simulink model "JKFF_CMOS"  (R2024b)
settings: Solver=VariableStepAuto  StartTime=0.0  StopTime=1e-6  RelTol=1e-3
libraries: ee_lib x22, fl_lib x10, nesl_utility x6
settings Model: Creator=Soochan Kim  LastModifiedBy=Soochan Kim

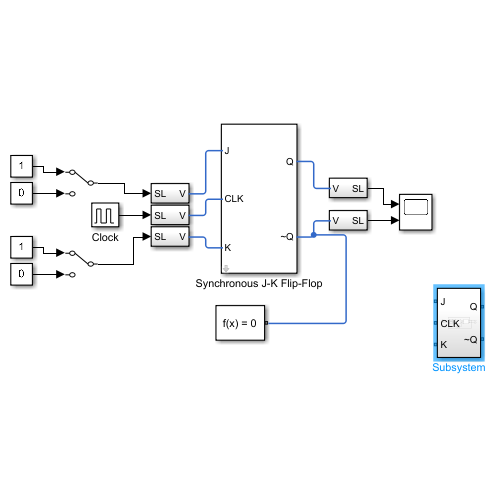
[thumbnail: Simulink's stored preview of the top-level diagram]
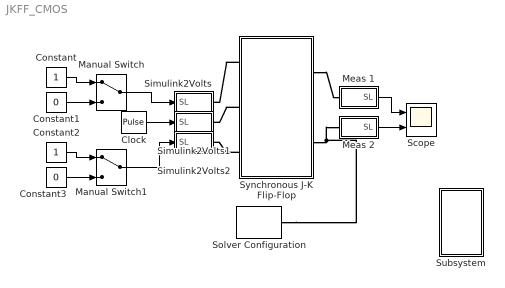
== system JKFF_CMOS ==
  Clock : DiscretePulseGenerator  PulseType=Time based  Amplitude=10  Period=2e-7  PulseWidth=50  PhaseDelay=0.5e-7
  Constant : Constant
  Constant1 : Constant  Value=0
  Constant2 : Constant
  Constant3 : Constant  Value=0
  Manual Switch : ManualSwitch
  Manual Switch1 : ManualSwitch
  Meas 1 : Subsystem
  Meas 2 : Subsystem
  Scope : Scope  NumInputPorts=2
  Simulink2Volts : Subsystem
  Simulink2Volts1 : Subsystem
  Simulink2Volts2 : Subsystem
  Solver Configuration : nesl_utility/Solver Configuration  PhysicalDomain=network_engine_domain  SubClassName=solver  LeftPortType=input  RightPortType=generic  Tones=[]  Harmonics=[]  SimulateNoise=off  Profile=off  UseLocalSampling=off  EnableSwitchedLinearOptims=on  FrequencyDomain=off  UseCCode=off  RelTol=0.001  AbsTol=0.001  MinStep=1e-09  ToWorkspace=off  RevertToSquareIcSolve=off  NumHomotopyIterations=100  PhasorMode=off  PhasorModeNumHarmonics=1  ConsistencySolver=NEWTON_XTOL_AFTER_FTOL  IndexReductionMethod=DerivativeReplacement  DoDC=off  ResidualTolerance=1e-09  ConsistencyTolSource=GLOBAL  ConsistencyAbsTol=0.001  ConsistencyRelTol=0.001  ConsistencyTolFactor=0.001  UseLocalSolver=off  LocalSolverChoice=NE_BACKWARD_EULER_ADVANCER  ResolveIndetEquations=on  FunctionEvalNumThread=1  LocalSolverSampleTime=0.001  DoFixedCost=off  MaxNonlinIter=3  MaxModeIter=2  ComputeImpulses=off  ImpulseIterations=2  LinearAlgebra=auto  LinearAlgebraNumThread=0  EquationFormulation=NE_TIME_EF  DelaysMemoryBudget=1024  AutomaticFiltering=on  FilteringTimeConstant=0.001  PartitionStorageMethod=AS_NEEDED  PartitionMemoryBudget=1024  PartitionMethod=ROBUST  MultibodyUseLocalSolver=off  MultibodyLocalSolverChoice=ODE1  MultibodyLocalSolverSampleTime=0.001
  Subsystem : Subsystem
  Synchronous J-K Flip-Flop : Subsystem  Tag=PublishSubsystem  mask(Synchronous J-K Flip-Flop){C_iss=0.1, t_p=1e-9, V_DD=10, R=450, state=High}
      mask prompts: C_iss "Gate input capacitance (pF)"; t_p "Gate propagation delay (s)"; V_DD "Supply voltage (V)"; R "Gate effective output resistance (ohms)"; state "Initial output"
      mask help: Behavioral model of a synchronous J-K flip-flop built from Simscape(TM) Electrical(TM) library components.
      mask init:
      | h = get_param(gcb,'Handle');
      | SR1 = sprintf('S-R Clocked\nFlip-Flop 1');
      | SR2 = sprintf('S-R Clocked\nFlip-Flop 2');
      | blk_path = [get_param(h,'Parent') '/' get_param(h,'Name')];
      | set_param([blk_path '/' SR1 '/NAND 3'],'output_state',num2str(state))
      | set_param([blk_path '/' SR2 '/NAND 3'],'output_state',num2str(state))
      | set_param([blk_path '/' SR1 '/NAND 4'],'output_state',num2str(3-state))
      | set_param([blk_path '/' SR2 '/NAND 4'],'output_state',num2str(3-state))
      mask TypeOptions state: Low | High
  wires:
  Constant/1 -> Manual Switch/1
  Constant1/1 -> Manual Switch/2
  Constant3/1 -> Manual Switch1/2
  Constant2/1 -> Manual Switch1/1
  Manual Switch/1 -> Simulink2Volts/1(SL)
  Manual Switch1/1 -> Simulink2Volts2/1(SL)
  Meas 1/1(SL) -> Scope/1
  Meas 2/1(SL) -> Scope/2
  Clock/1 -> Simulink2Volts1/1(SL)
  connections:
  Synchronous J-K Flip-Flop/RConn1 -- Meas 1/LConn1
  Synchronous J-K Flip-Flop/RConn2 -- Solver Configuration/RConn1 -- Meas 2/LConn1
  Synchronous J-K Flip-Flop/LConn1 -- Simulink2Volts/RConn1
  Synchronous J-K Flip-Flop/LConn2 -- Simulink2Volts1/RConn1
  Synchronous J-K Flip-Flop/LConn3 -- Simulink2Volts2/RConn1

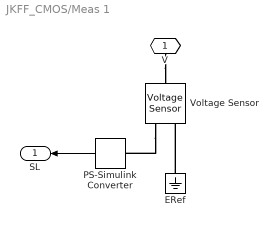
== system JKFF_CMOS/Meas 1 ==
  ERef : fl_lib/Electrical/Electrical Elements/Electrical Reference
  PS-Simulink Converter : nesl_utility/PS-Simulink Converter  PhysicalDomain=network_engine_domain  SubClassName=ps_output  LeftPortType=input  RightPortType=output  PseudoPeriodic=off  Frequencies=[]  VectorFormat=1-D array  Unit=V  AffineConversion=off
  Voltage Sensor : fl_lib/Electrical/Electrical Sensors/Voltage Sensor
  V : PMIOPort  Side=Left
  SL : Outport  VectorParamsAs1DForOutWhenUnconnected=off
  wires:
  PS-Simulink Converter/1 -> SL/1
  connections:
  V/RConn1 -- Voltage Sensor/LConn1
  ERef/LConn1 -- Voltage Sensor/RConn2
  Voltage Sensor/RConn1 -- PS-Simulink Converter/LConn1

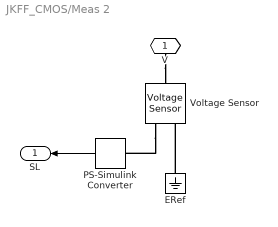
== system JKFF_CMOS/Meas 2 ==
  ERef : fl_lib/Electrical/Electrical Elements/Electrical Reference
  PS-Simulink Converter : nesl_utility/PS-Simulink Converter  PhysicalDomain=network_engine_domain  SubClassName=ps_output  LeftPortType=input  RightPortType=output  PseudoPeriodic=off  Frequencies=[]  VectorFormat=1-D array  Unit=V  AffineConversion=off
  Voltage Sensor : fl_lib/Electrical/Electrical Sensors/Voltage Sensor
  V : PMIOPort  Side=Left
  SL : Outport  VectorParamsAs1DForOutWhenUnconnected=off
  wires:
  PS-Simulink Converter/1 -> SL/1
  connections:
  V/RConn1 -- Voltage Sensor/LConn1
  ERef/LConn1 -- Voltage Sensor/RConn2
  Voltage Sensor/RConn1 -- PS-Simulink Converter/LConn1

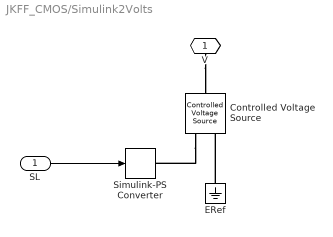
== system JKFF_CMOS/Simulink2Volts ==
  SL : Inport
  Controlled Voltage Source : fl_lib/Electrical/Electrical Sources/Controlled Voltage Source
  ERef : fl_lib/Electrical/Electrical Elements/Electrical Reference
  Simulink-PS Converter : nesl_utility/Simulink-PS Converter  PhysicalDomain=network_engine_domain  SubClassName=ps_input  LeftPortType=input  RightPortType=output  PseudoPeriodic=off  Frequencies=[]  NoiseDistribution=none  NoiseParameters=[]  Unit=V  AffineConversion=off  FilteringAndDerivatives=zero  SimscapeFilterOrder=1  InputFilterTimeConstant=.001  UdotUserProvided=0
  V : PMIOPort  Side=Right
  wires:
  SL/1 -> Simulink-PS Converter/1
  connections:
  V/RConn1 -- Controlled Voltage Source/LConn1
  ERef/LConn1 -- Controlled Voltage Source/RConn2
  Controlled Voltage Source/RConn1 -- Simulink-PS Converter/RConn1

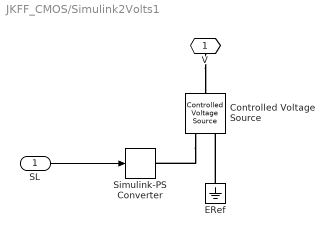
== system JKFF_CMOS/Simulink2Volts1 ==
  SL : Inport
  Controlled Voltage Source : fl_lib/Electrical/Electrical Sources/Controlled Voltage Source
  ERef : fl_lib/Electrical/Electrical Elements/Electrical Reference
  Simulink-PS Converter : nesl_utility/Simulink-PS Converter  PhysicalDomain=network_engine_domain  SubClassName=ps_input  LeftPortType=input  RightPortType=output  PseudoPeriodic=off  Frequencies=[]  NoiseDistribution=none  NoiseParameters=[]  Unit=V  AffineConversion=off  FilteringAndDerivatives=zero  SimscapeFilterOrder=1  InputFilterTimeConstant=.001  UdotUserProvided=0
  V : PMIOPort  Side=Right
  wires:
  SL/1 -> Simulink-PS Converter/1
  connections:
  V/RConn1 -- Controlled Voltage Source/LConn1
  ERef/LConn1 -- Controlled Voltage Source/RConn2
  Controlled Voltage Source/RConn1 -- Simulink-PS Converter/RConn1

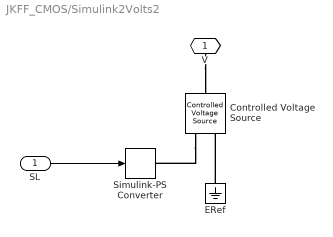
== system JKFF_CMOS/Simulink2Volts2 ==
  SL : Inport
  Controlled Voltage Source : fl_lib/Electrical/Electrical Sources/Controlled Voltage Source
  ERef : fl_lib/Electrical/Electrical Elements/Electrical Reference
  Simulink-PS Converter : nesl_utility/Simulink-PS Converter  PhysicalDomain=network_engine_domain  SubClassName=ps_input  LeftPortType=input  RightPortType=output  PseudoPeriodic=off  Frequencies=[]  NoiseDistribution=none  NoiseParameters=[]  Unit=V  AffineConversion=off  FilteringAndDerivatives=zero  SimscapeFilterOrder=1  InputFilterTimeConstant=.001  UdotUserProvided=0
  V : PMIOPort  Side=Right
  wires:
  SL/1 -> Simulink-PS Converter/1
  connections:
  V/RConn1 -- Controlled Voltage Source/LConn1
  ERef/LConn1 -- Controlled Voltage Source/RConn2
  Controlled Voltage Source/RConn1 -- Simulink-PS Converter/RConn1

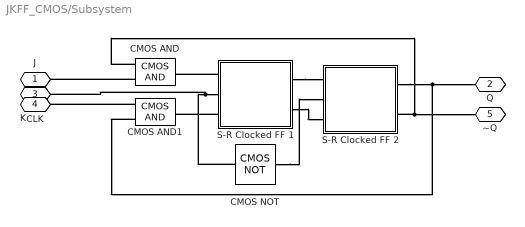
== system JKFF_CMOS/Subsystem ==
  CMOS AND : ee_lib/Integrated Circuits/Logic/CMOS AND  V_IL=2 V  V_IH=3 V  C_IN=5 pF  output_type=ee.enum.ic.outputType.linear  V_OL=0 V  V_OH=5 V  V_CC=5 V  V_meas=5 V  R_OUT=25 Ohm  R_OH=[25, 250] Ohm  I_OH=63 mA  R_OL=[30, 800] Ohm  I_OL=-45 mA  Delay=25 ns  Ron=5 Ohm  Vf=0.6 V  output_state=ee.enum.ic.initialState.low
      settings: InternalSimscapePortConfiguration="{\"Bottom\":[],\"Left\":[{\"id\":\"A\",\"label\":\"\",\"type\":\"foundation.electrical.electrical\"},{\"id\":\"B\",\"label\":\"\",\"type\":\"foundation.electrical.electrical\"}],\"Right\":[{\"id\":\"J\",\"label\":\"\",\"type\":\"foundation.electrical.electrical\"}],\"Top\":[]}"
  CMOS AND1 : ee_lib/Integrated Circuits/Logic/CMOS AND  V_IL=2 V  V_IH=3 V  C_IN=5 pF  output_type=ee.enum.ic.outputType.linear  V_OL=0 V  V_OH=5 V  V_CC=5 V  V_meas=5 V  R_OUT=25 Ohm  R_OH=[25, 250] Ohm  I_OH=63 mA  R_OL=[30, 800] Ohm  I_OL=-45 mA  Delay=25 ns  Ron=5 Ohm  Vf=0.6 V  output_state=ee.enum.ic.initialState.low
      settings: InternalSimscapePortConfiguration="{\"Bottom\":[],\"Left\":[{\"id\":\"A\",\"label\":\"\",\"type\":\"foundation.electrical.electrical\"},{\"id\":\"B\",\"label\":\"\",\"type\":\"foundation.electrical.electrical\"}],\"Right\":[{\"id\":\"J\",\"label\":\"\",\"type\":\"foundation.electrical.electrical\"}],\"Top\":[]}"
  CMOS NOT : ee_lib/Integrated Circuits/Logic/CMOS NOT  V_IL=2 V  V_IH=3 V  C_IN=5 pF  output_type=ee.enum.ic.outputType.linear  V_OL=0 V  V_OH=5 V  V_CC=5 V  V_meas=5 V  R_OUT=25 Ohm  R_OH=[25, 250] Ohm  I_OH=63 mA  R_OL=[30, 800] Ohm  I_OL=-45 mA  Delay=25 ns  Ron=5 Ohm  Vf=0.6 V  output_state=ee.enum.ic.initialState.low
      settings: InternalSimscapePortConfiguration="{\"Bottom\":[],\"Left\":[{\"id\":\"A\",\"label\":\"\",\"type\":\"foundation.electrical.electrical\"}],\"Right\":[{\"id\":\"J\",\"label\":\"\",\"type\":\"foundation.electrical.electrical\"}],\"Top\":[]}"
  S-R Clocked FF 1 : Subsystem
  S-R Clocked FF 2 : Subsystem
  J : PMIOPort  Side=Left
  Q : PMIOPort  Port=2  Side=Right
  CLK : PMIOPort  Port=3  Side=Left
  K : PMIOPort  Port=4  Side=Left
  ~Q : PMIOPort  Port=5  Side=Right
  connections:
  CMOS AND/LConn1 -- S-R Clocked FF 2/RConn2 -- ~Q/RConn1
  S-R Clocked FF 1/LConn3 -- CMOS AND1/RConn1
  S-R Clocked FF 1/RConn1 -- S-R Clocked FF 2/LConn1
  S-R Clocked FF 1/RConn2 -- S-R Clocked FF 2/LConn3
  CMOS NOT/RConn1 -- S-R Clocked FF 2/LConn2
  CMOS AND1/LConn2 -- S-R Clocked FF 2/RConn1 -- Q/RConn1
  CMOS AND1/LConn1 -- K/RConn1
  S-R Clocked FF 1/LConn1 -- CMOS AND/RConn1
  S-R Clocked FF 1/LConn2 -- CMOS NOT/LConn1 -- CLK/RConn1
  CMOS AND/LConn2 -- J/RConn1

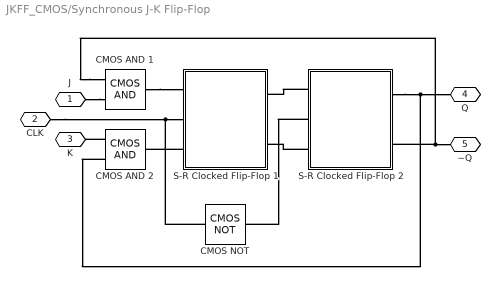
== system JKFF_CMOS/Synchronous J-K Flip-Flop ==
  CMOS AND 1 : ee_lib/Integrated Circuits/Logic/CMOS AND  V_IL=0.4*V_DD V  V_IH=0.6*V_DD V  C_IN=C_iss pF  output_type=1  V_OL=0 V  V_OH=V_DD V  V_CC=5 V  V_meas=5 V  R_OUT=R Ohm  R_OH=[ 25 250 ] Ohm  I_OH=63 mA  R_OL=[ 30 800 ] Ohm  I_OL=-45 mA  Delay=t_p s  Ron=5 Ohm  Vf=0.6 V  output_state=1
      settings: InternalSimscapePortConfiguration="{\"Bottom\":[],\"Left\":[{\"id\":\"A\",\"label\":\"\",\"type\":\"foundation.electrical.electrical\"},{\"id\":\"B\",\"label\":\"\",\"type\":\"foundation.electrical.electrical\"}],\"Right\":[{\"id\":\"J\",\"label\":\"\",\"type\":\"foundation.electrical.electrical\"}],\"Top\":[]}"
  CMOS AND 2 : ee_lib/Integrated Circuits/Logic/CMOS AND  V_IL=0.4*V_DD V  V_IH=0.6*V_DD V  C_IN=C_iss pF  output_type=1  V_OL=0 V  V_OH=V_DD V  V_CC=5 V  V_meas=5 V  R_OUT=R Ohm  R_OH=[ 25 250 ] Ohm  I_OH=63 mA  R_OL=[ 30 800 ] Ohm  I_OL=-45 mA  Delay=t_p s  Ron=5 Ohm  Vf=0.6 V  output_state=1
      settings: InternalSimscapePortConfiguration="{\"Bottom\":[],\"Left\":[{\"id\":\"A\",\"label\":\"\",\"type\":\"foundation.electrical.electrical\"},{\"id\":\"B\",\"label\":\"\",\"type\":\"foundation.electrical.electrical\"}],\"Right\":[{\"id\":\"J\",\"label\":\"\",\"type\":\"foundation.electrical.electrical\"}],\"Top\":[]}"
  CMOS NOT : ee_lib/Integrated Circuits/Logic/CMOS NOT  V_IL=0.4*V_DD V  V_IH=0.6*V_DD V  C_IN=C_iss pF  output_type=1  V_OL=0 V  V_OH=V_DD V  V_CC=5 V  V_meas=5 V  R_OUT=R Ohm  R_OH=[ 25 250 ] Ohm  I_OH=63 mA  R_OL=[ 30 800 ] Ohm  I_OL=-45 mA  Delay=t_p s  Ron=5 Ohm  Vf=0.6 V  output_state=1
      settings: InternalSimscapePortConfiguration="{\"Bottom\":[],\"Left\":[{\"id\":\"A\",\"label\":\"\",\"type\":\"foundation.electrical.electrical\"}],\"Right\":[{\"id\":\"J\",\"label\":\"\",\"type\":\"foundation.electrical.electrical\"}],\"Top\":[]}"
  S-R Clocked Flip-Flop 1 : Subsystem  Tag=PublishSubsystem
  S-R Clocked Flip-Flop 2 : Subsystem
  J : PMIOPort  Side=Left
  CLK : PMIOPort  Port=2  Side=Left
  K : PMIOPort  Port=3  Side=Left
  Q : PMIOPort  Port=4  Side=Right
  ~Q : PMIOPort  Port=5  Side=Right
  connections:
  S-R Clocked Flip-Flop 2/LConn2 -- CMOS NOT/RConn1
  S-R Clocked Flip-Flop 2/LConn1 -- S-R Clocked Flip-Flop 1/RConn1
  S-R Clocked Flip-Flop 2/LConn3 -- S-R Clocked Flip-Flop 1/RConn2
  CMOS AND 2/LConn2 -- S-R Clocked Flip-Flop 2/RConn1 -- Q/RConn1
  CMOS AND 1/LConn1 -- ~Q/RConn1 -- S-R Clocked Flip-Flop 2/RConn2
  J/RConn1 -- CMOS AND 1/LConn2
  CMOS AND 1/RConn1 -- S-R Clocked Flip-Flop 1/LConn1
  CMOS AND 2/LConn1 -- K/RConn1
  S-R Clocked Flip-Flop 1/LConn3 -- CMOS AND 2/RConn1
  CLK/RConn1 -- CMOS NOT/LConn1 -- S-R Clocked Flip-Flop 1/LConn2

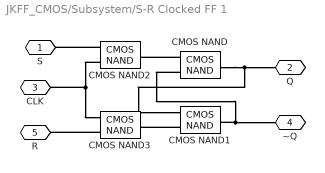
== system JKFF_CMOS/Subsystem/S-R Clocked FF 1 ==
  CMOS NAND{,1..3} (4 alike) : ee_lib/Integrated Circuits/Logic/CMOS NAND  V_IL=2 V  V_IH=3 V  C_IN=5 pF  output_type=ee.enum.ic.outputType.linear  V_OL=0 V  V_OH=5 V  V_CC=5 V  V_meas=5 V  R_OUT=25 Ohm  R_OH=[25, 250] Ohm  I_OH=63 mA  R_OL=[30, 800] Ohm  I_OL=-45 mA  Delay=25 ns  Ron=5 Ohm  Vf=0.6 V  output_state=ee.enum.ic.initialState.low
      settings: InternalSimscapePortConfiguration="{\"Bottom\":[],\"Left\":[{\"id\":\"A\",\"label\":\"\",\"type\":\"foundation.electrical.electrical\"},{\"id\":\"B\",\"label\":\"\",\"type\":\"foundation.electrical.electrical\"}],\"Right\":[{\"id\":\"J\",\"label\":\"\",\"type\":\"foundation.electrical.electrical\"}],\"Top\":[]}"
  S : PMIOPort  Side=Left
  Q : PMIOPort  Port=2  Side=Right
  CLK : PMIOPort  Port=3  Side=Left
  ~Q : PMIOPort  Port=4  Side=Right
  R : PMIOPort  Port=5  Side=Left
  connections:
  CMOS NAND1/LConn2 -- CMOS NAND3/RConn1
  CMOS NAND/LConn2 -- CMOS NAND1/RConn1 -- ~Q/RConn1
  CMOS NAND/RConn1 -- CMOS NAND1/LConn1 -- Q/RConn1
  CMOS NAND3/LConn2 -- R/RConn1
  CMOS NAND2/LConn2 -- CLK/RConn1 -- CMOS NAND3/LConn1
  CMOS NAND2/LConn1 -- S/RConn1
  CMOS NAND/LConn1 -- CMOS NAND2/RConn1

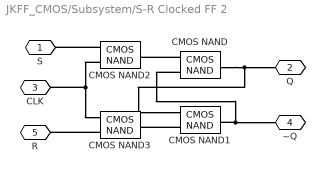
== system JKFF_CMOS/Subsystem/S-R Clocked FF 2 ==
  CMOS NAND{,1..3} (4 alike) : ee_lib/Integrated Circuits/Logic/CMOS NAND  V_IL=2 V  V_IH=3 V  C_IN=5 pF  output_type=ee.enum.ic.outputType.linear  V_OL=0 V  V_OH=5 V  V_CC=5 V  V_meas=5 V  R_OUT=25 Ohm  R_OH=[25, 250] Ohm  I_OH=63 mA  R_OL=[30, 800] Ohm  I_OL=-45 mA  Delay=25 ns  Ron=5 Ohm  Vf=0.6 V  output_state=ee.enum.ic.initialState.low
      settings: InternalSimscapePortConfiguration="{\"Bottom\":[],\"Left\":[{\"id\":\"A\",\"label\":\"\",\"type\":\"foundation.electrical.electrical\"},{\"id\":\"B\",\"label\":\"\",\"type\":\"foundation.electrical.electrical\"}],\"Right\":[{\"id\":\"J\",\"label\":\"\",\"type\":\"foundation.electrical.electrical\"}],\"Top\":[]}"
  S : PMIOPort  Side=Left
  Q : PMIOPort  Port=2  Side=Right
  CLK : PMIOPort  Port=3  Side=Left
  ~Q : PMIOPort  Port=4  Side=Right
  R : PMIOPort  Port=5  Side=Left
  connections:
  CMOS NAND1/LConn2 -- CMOS NAND3/RConn1
  CMOS NAND/LConn2 -- CMOS NAND1/RConn1 -- ~Q/RConn1
  CMOS NAND/RConn1 -- CMOS NAND1/LConn1 -- Q/RConn1
  CMOS NAND3/LConn2 -- R/RConn1
  CMOS NAND2/LConn2 -- CLK/RConn1 -- CMOS NAND3/LConn1
  CMOS NAND2/LConn1 -- S/RConn1
  CMOS NAND/LConn1 -- CMOS NAND2/RConn1

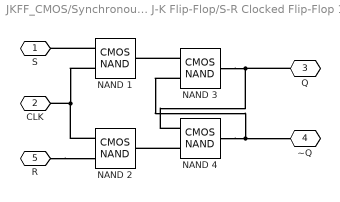
== system JKFF_CMOS/Synchronous J-K Flip-Flop/S-R Clocked Flip-Flop 1 ==
  NAND 1 : ee_lib/Integrated Circuits/Logic/CMOS NAND  V_IL=0.4*V_DD V  V_IH=0.6*V_DD V  C_IN=C_iss pF  output_type=1  V_OL=0 V  V_OH=V_DD V  V_CC=5 V  V_meas=5 V  R_OUT=R Ohm  R_OH=[ 25 250 ] Ohm  I_OH=63 mA  R_OL=[ 30 800 ] Ohm  I_OL=-45 mA  Delay=t_p s  Ron=5 Ohm  Vf=0.6 V  output_state=1
      settings: InternalSimscapePortConfiguration="{\"Bottom\":[],\"Left\":[{\"id\":\"A\",\"label\":\"\",\"type\":\"foundation.electrical.electrical\"},{\"id\":\"B\",\"label\":\"\",\"type\":\"foundation.electrical.electrical\"}],\"Right\":[{\"id\":\"J\",\"label\":\"\",\"type\":\"foundation.electrical.electrical\"}],\"Top\":[]}"
  NAND 2 : ee_lib/Integrated Circuits/Logic/CMOS NAND  V_IL=0.4*V_DD V  V_IH=0.6*V_DD V  C_IN=C_iss pF  output_type=1  V_OL=0 V  V_OH=V_DD V  V_CC=5 V  V_meas=5 V  R_OUT=R Ohm  R_OH=[ 25 250 ] Ohm  I_OH=63 mA  R_OL=[ 30 800 ] Ohm  I_OL=-45 mA  Delay=t_p s  Ron=5 Ohm  Vf=0.6 V  output_state=1
      settings: InternalSimscapePortConfiguration="{\"Bottom\":[],\"Left\":[{\"id\":\"A\",\"label\":\"\",\"type\":\"foundation.electrical.electrical\"},{\"id\":\"B\",\"label\":\"\",\"type\":\"foundation.electrical.electrical\"}],\"Right\":[{\"id\":\"J\",\"label\":\"\",\"type\":\"foundation.electrical.electrical\"}],\"Top\":[]}"
  NAND 3 : ee_lib/Integrated Circuits/Logic/CMOS NAND  V_IL=0.4*V_DD V  V_IH=0.6*V_DD V  C_IN=C_iss pF  output_type=1  V_OL=0 V  V_OH=V_DD V  V_CC=5 V  V_meas=5 V  R_OUT=R Ohm  R_OH=[ 25 250 ] Ohm  I_OH=63 mA  R_OL=[ 30 800 ] Ohm  I_OL=-45 mA  Delay=t_p s  Ron=5 Ohm  Vf=0.6 V  output_state=2
      settings: InternalSimscapePortConfiguration="{\"Bottom\":[],\"Left\":[{\"id\":\"A\",\"label\":\"\",\"type\":\"foundation.electrical.electrical\"},{\"id\":\"B\",\"label\":\"\",\"type\":\"foundation.electrical.electrical\"}],\"Right\":[{\"id\":\"J\",\"label\":\"\",\"type\":\"foundation.electrical.electrical\"}],\"Top\":[]}"
  NAND 4 : ee_lib/Integrated Circuits/Logic/CMOS NAND  V_IL=0.4*V_DD V  V_IH=0.6*V_DD V  C_IN=C_iss pF  output_type=1  V_OL=0 V  V_OH=V_DD V  V_CC=5 V  V_meas=5 V  R_OUT=R Ohm  R_OH=[ 25 250 ] Ohm  I_OH=63 mA  R_OL=[ 30 800 ] Ohm  I_OL=-45 mA  Delay=t_p s  Ron=5 Ohm  Vf=0.6 V  output_state=1
      settings: InternalSimscapePortConfiguration="{\"Bottom\":[],\"Left\":[{\"id\":\"A\",\"label\":\"\",\"type\":\"foundation.electrical.electrical\"},{\"id\":\"B\",\"label\":\"\",\"type\":\"foundation.electrical.electrical\"}],\"Right\":[{\"id\":\"J\",\"label\":\"\",\"type\":\"foundation.electrical.electrical\"}],\"Top\":[]}"
  S : PMIOPort  Side=Left
  CLK : PMIOPort  Port=2  Side=Left
  Q : PMIOPort  Port=3  Side=Right
  ~Q : PMIOPort  Port=4  Side=Right
  R : PMIOPort  Port=5  Side=Left
  connections:
  NAND 2/LConn1 -- CLK/RConn1 -- NAND 1/LConn2
  NAND 3/LConn1 -- NAND 1/RConn1
  NAND 4/LConn2 -- NAND 2/RConn1
  NAND 4/RConn1 -- ~Q/RConn1 -- NAND 3/LConn2
  NAND 4/LConn1 -- Q/RConn1 -- NAND 3/RConn1
  NAND 1/LConn1 -- S/RConn1
  R/RConn1 -- NAND 2/LConn2

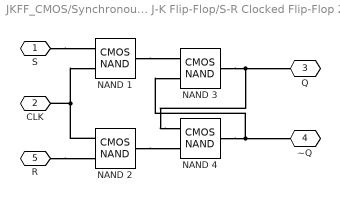
== system JKFF_CMOS/Synchronous J-K Flip-Flop/S-R Clocked Flip-Flop 2 ==
  NAND 1 : ee_lib/Integrated Circuits/Logic/CMOS NAND  V_IL=0.4*V_DD V  V_IH=0.6*V_DD V  C_IN=C_iss pF  output_type=1  V_OL=0 V  V_OH=V_DD V  V_CC=5 V  V_meas=5 V  R_OUT=R Ohm  R_OH=[ 25 250 ] Ohm  I_OH=63 mA  R_OL=[ 30 800 ] Ohm  I_OL=-45 mA  Delay=t_p s  Ron=5 Ohm  Vf=0.6 V  output_state=1
      settings: InternalSimscapePortConfiguration="{\"Bottom\":[],\"Left\":[{\"id\":\"A\",\"label\":\"\",\"type\":\"foundation.electrical.electrical\"},{\"id\":\"B\",\"label\":\"\",\"type\":\"foundation.electrical.electrical\"}],\"Right\":[{\"id\":\"J\",\"label\":\"\",\"type\":\"foundation.electrical.electrical\"}],\"Top\":[]}"
  NAND 2 : ee_lib/Integrated Circuits/Logic/CMOS NAND  V_IL=0.4*V_DD V  V_IH=0.6*V_DD V  C_IN=C_iss pF  output_type=1  V_OL=0 V  V_OH=V_DD V  V_CC=5 V  V_meas=5 V  R_OUT=R Ohm  R_OH=[ 25 250 ] Ohm  I_OH=63 mA  R_OL=[ 30 800 ] Ohm  I_OL=-45 mA  Delay=t_p s  Ron=5 Ohm  Vf=0.6 V  output_state=1
      settings: InternalSimscapePortConfiguration="{\"Bottom\":[],\"Left\":[{\"id\":\"A\",\"label\":\"\",\"type\":\"foundation.electrical.electrical\"},{\"id\":\"B\",\"label\":\"\",\"type\":\"foundation.electrical.electrical\"}],\"Right\":[{\"id\":\"J\",\"label\":\"\",\"type\":\"foundation.electrical.electrical\"}],\"Top\":[]}"
  NAND 3 : ee_lib/Integrated Circuits/Logic/CMOS NAND  V_IL=0.4*V_DD V  V_IH=0.6*V_DD V  C_IN=C_iss pF  output_type=1  V_OL=0 V  V_OH=V_DD V  V_CC=5 V  V_meas=5 V  R_OUT=R Ohm  R_OH=[ 25 250 ] Ohm  I_OH=63 mA  R_OL=[ 30 800 ] Ohm  I_OL=-45 mA  Delay=t_p s  Ron=5 Ohm  Vf=0.6 V  output_state=2
      settings: InternalSimscapePortConfiguration="{\"Bottom\":[],\"Left\":[{\"id\":\"A\",\"label\":\"\",\"type\":\"foundation.electrical.electrical\"},{\"id\":\"B\",\"label\":\"\",\"type\":\"foundation.electrical.electrical\"}],\"Right\":[{\"id\":\"J\",\"label\":\"\",\"type\":\"foundation.electrical.electrical\"}],\"Top\":[]}"
  NAND 4 : ee_lib/Integrated Circuits/Logic/CMOS NAND  V_IL=0.4*V_DD V  V_IH=0.6*V_DD V  C_IN=C_iss pF  output_type=1  V_OL=0 V  V_OH=V_DD V  V_CC=5 V  V_meas=5 V  R_OUT=R Ohm  R_OH=[ 25 250 ] Ohm  I_OH=63 mA  R_OL=[ 30 800 ] Ohm  I_OL=-45 mA  Delay=t_p s  Ron=5 Ohm  Vf=0.6 V  output_state=1
      settings: InternalSimscapePortConfiguration="{\"Bottom\":[],\"Left\":[{\"id\":\"A\",\"label\":\"\",\"type\":\"foundation.electrical.electrical\"},{\"id\":\"B\",\"label\":\"\",\"type\":\"foundation.electrical.electrical\"}],\"Right\":[{\"id\":\"J\",\"label\":\"\",\"type\":\"foundation.electrical.electrical\"}],\"Top\":[]}"
  S : PMIOPort  Side=Left
  CLK : PMIOPort  Port=2  Side=Left
  Q : PMIOPort  Port=3  Side=Right
  ~Q : PMIOPort  Port=4  Side=Right
  R : PMIOPort  Port=5  Side=Left
  connections:
  R/RConn1 -- NAND 2/LConn2
  S/RConn1 -- NAND 1/LConn1
  NAND 4/LConn1 -- Q/RConn1 -- NAND 3/RConn1
  NAND 4/RConn1 -- ~Q/RConn1 -- NAND 3/LConn2
  NAND 2/RConn1 -- NAND 4/LConn2
  NAND 1/RConn1 -- NAND 3/LConn1
  NAND 2/LConn1 -- CLK/RConn1 -- NAND 1/LConn2
